simulink model "Project_P35_1"  (R2021b)
settings: Solver=VariableStepAuto  StartTime=0.0  StopTime=10.0  RelTol=1e-3
settings Model: Creator=yingguang wang  LastModifiedBy=yingguang wang

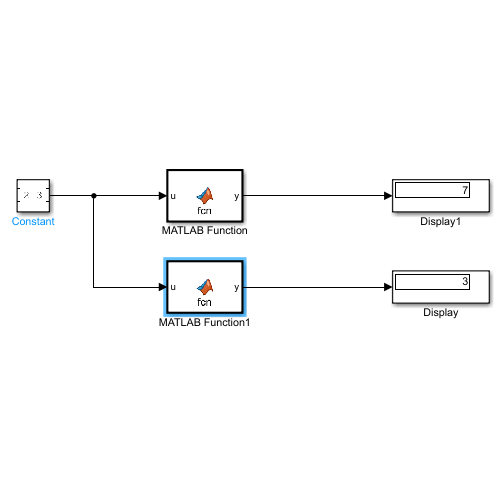
[thumbnail: Simulink's stored preview of the top-level diagram]
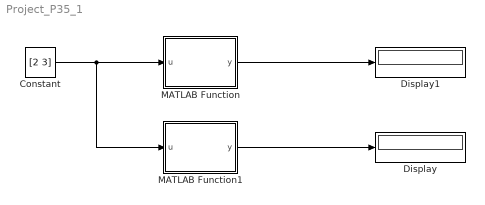
== system Project_P35_1 ==
  Constant : Constant  Value=[2 3]
  Display : Display
  Display1 : Display
  MATLAB Function : MATLAB Function  TreatAsAtomicUnit=on
  MATLAB Function1 : MATLAB Function  TreatAsAtomicUnit=on
  wires:
  Constant/1 -> MATLAB Function1/1(u), MATLAB Function/1(u)
  MATLAB Function1/1(y) -> Display/1
  MATLAB Function/1(y) -> Display1/1

== matlab function Project_P35_1/MATLAB Function ==
  data: u input; y output
function y = fcn(u)

y = u(1)*u(1)+u(2);

== matlab function Project_P35_1/MATLAB Function1 ==
  data: u input; y output
function y = fcn(u)

y = max(u(1),u(2));
